simulink library "dsparch2"  (Simulink 3.00)
values from neighbouring files (symbols this model uses):
  h = h./max(h)*0.75    [dspfdes.m]    (also in dspfwiz.m = fdatool(opts); sdspfscope.m = fig_data.menu.memory)
undefined symbols (not defined in the file or in its folder): fchans
libraries: dspbuff2 x4, dspxfrm2 x4, dspbdsp2 x1
settings Model: Creator=szlotkin  LastModifiedBy=jeff

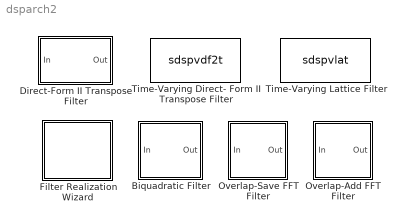
== system dsparch2 ==
  Biquadratic Filter : Subsystem  mask(Biquadratic Filter){sos=[0.0864663705046504 0.172963265055902 0.0864691222801249 1 -0.835073472386969 0.180972230227646;0.0910631887324868 0.184433970597206 0.0934004367730367 1 -0.890597579638043 0.259495175740772;0.10515199960233 0.210266887507767 0.105148652679738 1 -1.0153398584545 0.43590739824434;0.13033445611126 0.257366152017378 0.127072973655515 1 -1.24277336269468 0.75754694447883], ic=0, frame=off, nchans=1}
      mask prompts: sos "SOS matrix:"; ic "Initial conditions:"; frame "Frame-based inputs"; nchans "Number of channels:"
      mask help:
      | Direct-Form II Transpose implementation of second-order (biquadratic) IIR filter sections.  Coefficients must be expressed using an Mx6 second-order section (SOS) matrix.  The number of second-order sections (M) appears in the lower-right corner of the icon.
      |
      | See "ss2sos" for more information on SOS matrices.
      mask init:
      | [x,y,s]=dspblkbiquad('icon',sos);
      | [h,fchans]=dspblkbiquad('init',sos,frame,nchans);
      mask Help: web(dspbhelp);
      mask CallbackString: ||dspblkbiquad|
      mask Display:
      | plot(x,y);
      | text(.975,0.1,s,'horiz','right');
      | text(0.1,.9,'BiQuad')
  Direct-Form II Transpose Filter : Subsystem  mask(Direct-Form II Transpose Filter){num=[1 2], den=1, ic=0, frame=off, numCHANS=1}
      mask prompts: num "Numerator:"; den "Denominator:"; ic "Initial conditions:"; frame "Frame-based inputs"; numCHANS "Number of channels:"
      mask help:
      | Independently filters each channel of input over time using a Direct-Form II Transpose  implementation.  Initial conditions are interpreted in the same manner as MATLAB's "filter" command.
      |
      | For frame-based processing, each column of the input matrix represents one frame of data from a single channel.
      mask init:
      | [x,y] = dspblkdf2t('icon',num,den);
      | if strcmp(frame,'off'), numCHANS=-1; end
      | [num,den] = dspblkdf2t('design',num,den);
      mask Help: web(dspbhelp);
      mask CallbackString: |||dspblkdf2t|
      mask Display:
      | plot(x,y);
      | text(0.5,.85,'DF2T','horiz','center');
  Filter Realization Wizard : Subsystem  mask(Filter Realization Wizard){}
      mask help: Automatically construct filter realizations with specific architectures, using sum, gain, and delay blocks.
      mask init:
      | xw=[NaN 0.8 0.8 NaN 0.687 0.743 NaN 0.64 0.72 NaN 0.687 0.743 NaN 0.8 0.8 NaN 0.913 0.857 NaN 0.96 0.88 NaN 0.808 0.792 0.961 0.978 0.808 NaN 0.825 0.808 NaN 0.961 0.944];
      | yw=[NaN 0.64 0.72 NaN 0.687 0.743 NaN 0.8 0.8 NaN 0.913 0.857 NaN 0.96 0.88 NaN 0.913 0.857 NaN 0.8 0.8 NaN 0.808 0.792 0.622 0.639 0.808 NaN 0.792 0.775 NaN 0.656 0.639];
      | 
      | xl = [.1 .7 NaN .3 .3 NaN .7 .7 NaN .3 .3 NaN .7 .7 NaN .3 .9];
      | yl = [.8 .8 NaN .8 .6 NaN .8 .6 NaN .4 .2 NaN .4 .13 NaN .2 .2];
      | xz = [.46 .54 .46 NaN .54 .59 .54 .59 NaN .61 .64 NaN .67 .67];
      | yz = [.84 .8  .76 NaN .92 .92 .86 .86 NaN .93 .93 NaN .97 .89];
      | xg = [.21 .39 .3 .21 NaN .61 .79 .7 .61];
      | yg = [.6  .6  .4 .6  NaN .6  .6  .4 .6];
      | t=(0:12)/12*2*pi;
      | xs = .07*cos(t)+.7;
      | ys = .07*sin(t)+.2;
      settings: OpenFcn=dspfwiz
      mask Help: web(dspbhelp);
      mask Display:
      | plot([[xl NaN xz NaN xg NaN xs NaN]*.9-.075 xw],
      | [[yl NaN yz NaN yg NaN ys NaN]*.9-.1 yw]);
  Overlap-Add FFT Filter : Subsystem  mask(Overlap-Add FFT Filter){Nfft=64, h=fir1(20,0.1)}
      mask prompts: Nfft "FFT size:"; h "FIR coefficients:"
      mask help: FFT based filtering using the overlap-add algorithm.
      mask init:
      | M = length(h); N=2.^nextpow2(Nfft); L=N-M+1;
      | H = freqz(h,1,N,'whole');
      mask Help: web(dspbhelp);
      mask Display:
      | disp('Overlap\nAdd');
      | ... plot(log10(abs(H(1:(N/2)))))
  Overlap-Save FFT Filter : Subsystem  mask(Overlap-Save FFT Filter){nfft_in=64, h=fir1(20,0.1)}
      mask prompts: nfft_in "FFT size:"; h "FIR coefficients:"
      mask help: FFT based filtering using the overlap-save algorithm.
      mask init:
      | nfft = 2.^nextpow2(nfft_in);
      | n = length(h); H = freqz(h,1,nfft,'whole');
      mask Help: web(dspbhelp);
      mask Display:
      | disp('Overlap\nSave');
      | ... plot(log10(abs(H(1:(nfft/2)))))
  Time-Varying Lattice Filter : S-Function  FunctionName=sdspvlat  Parameters=ARMA, ic, numCHANS, FiltPerFrame  PortCounts=[]  SFunctionModules=''  mask(Time-Varying Lattice Filter){ARMA=All-Zero (MA), ic=0, frame=off, numCHANS=1, FiltPerFrame=One Filter Per Sample Time}
      mask prompts: ARMA "Filter type:"; ic "Initial conditions:"; frame "Frame-based inputs"; numCHANS "Number of channels:"; FiltPerFrame "Filter update rate:"
      mask help:
      | Independently filters each channel of input over time using a Lattice implementation.  Filter coefficients can vary over time.
      |
      | For frame-based processing, multiple data channels may be passed as a frame matrix, with one channel per column.  The filter update rate is selectable.
      mask init:
      | [x,y,s] = dspblkvlat(ARMA);
      | if strcmp(frame,'off') numCHANS = -1; end
      mask Help: web(dspbhelp);
      mask StyleString: popup(All-Zero (MA)|All-Pole (AR)),edit,checkbox,edit,popup(One Filter Per Sample Time|One Filter Per Frame Time)
      mask CallbackString: ||dspblkvlat||
      mask Display:
      | plot(x,y);
      | port_label('input',1,'In');
      | port_label('output',1,'Out');
      | port_label('input',s.i1,s.s1);
      | port_label('input',s.i2,s.s2);
  Time-Varying Direct- Form II Transpose Filter : S-Function  FunctionName=sdspvdf2t  Parameters=NumDen, ic, filtCheck,numCHANS, FiltPerFrame  PortCounts=[]  SFunctionModules=''  mask(Time-Varying Direct-Form II Transpose Filter){NumDen=Pole-Zero (IIR), ic=0, filtCheck=on, frame=off, numCHANS=1, FiltPerFrame=One Filter Per Sample Time}
      mask prompts: NumDen "Filter type:"; ic "Initial conditions:"; filtCheck "Support non-normalized filters"; frame "Frame-based inputs"; numCHANS "Number of channels:"; FiltPerFrame "Filter update rate:"
      mask help:
      | Independently filters each channel of input over time using a Direct-Form II Transpose implementation.  Filter coefficients can vary over time.
      |
      | Initial conditions are interpreted in the same manner as MATLAB's "filter" command.  However, this time-varying filter uses a different normalization scheme and the initial conditions and internal filter states are not equivalent to those from "filter" if the first denominator coefficient is not 1.0.   If "Support non-normalized filters" is deselected, the leading denominator coefficient is assumed to be 1.0.
      |
      | For frame-based processing, multiple data channels may be passed as a frame matrix, with one channel per column.  The filter update rate is selectable.
      mask init:
      | s = dspblkvdf2t(NumDen);
      | if strcmp(frame,'off') numCHANS = -1; end
      mask Help: web(dspbhelp);
      mask StyleString: popup(Pole-Zero (IIR)|All-Zero (FIR)|All-Pole (AR)),edit,checkbox,checkbox,edit,popup(One Filter Per Sample Time|One Filter Per Frame Time)
      mask CallbackString: |||dspblkvdf2t||
      mask Display:
      | text(0.5,0.85,s.icon,'horiz','center');
      | plot(s.x, s.y);
      | port_label('input',1,'In');
      | port_label('output',1,'Out');
      | port_label('input',s.i1,s.s1);
      | port_label('input',s.i2,s.s2);

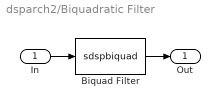
== system dsparch2/Biquadratic Filter ==
  In : Inport  Port=1  PortWidth=-1  SampleTime=-1  DataType=auto
      settings: SignalType=auto
  Biquad Filter : S-Function  FunctionName=sdspbiquad  Parameters=h,ic,fchans  PortCounts=[]  SFunctionModules=''
  Out : Outport  Port=1  InitialOutput=0
  wires:
  In/1 -> Biquad Filter/1
  Biquad Filter/1 -> Out/1

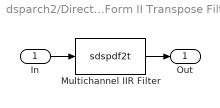
== system dsparch2/Direct-Form II Transpose Filter ==
  In : Inport  Port=1  PortWidth=-1  SampleTime=-1  DataType=auto
      settings: SignalType=auto
  Multichannel IIR Filter : S-Function  FunctionName=sdspdf2t  Parameters=num,den,ic,numCHANS  PortCounts=[]  SFunctionModules=''
  Out : Outport  Port=1  InitialOutput=0
  wires:
  Multichannel IIR Filter/1 -> Out/1
  In/1 -> Multichannel IIR Filter/1

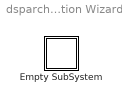
== system dsparch2/Filter Realization Wizard ==
  Empty SubSystem : Subsystem

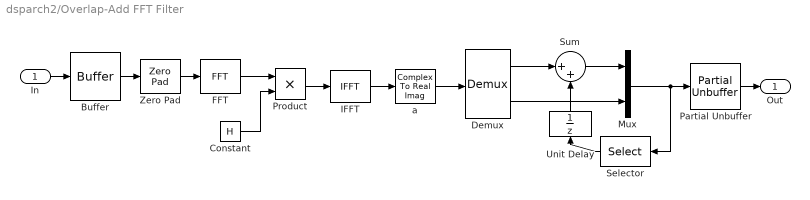
== system dsparch2/Overlap-Add FFT Filter ==
  In : Inport  Port=1  PortWidth=-1  SampleTime=-1  DataType=auto
      settings: SignalType=auto
  Buffer : dspbuff2/Buffer  N=L  V=0  ic=0
  Constant : Constant  Value=H
  Demux : Demux  Outputs=[M-1 L]
  FFT : dspxfrm2/FFT  nchans=1
  IFFT : dspxfrm2/IFFT  mode=Complex  cs_in=off  nchans=1
  Mux : Mux  Inputs=2
  Partial Unbuffer : dspbuff2/Partial Unbuffer  N=N  N1=1  N2=L  ic=0  num_chans=1
  Product : Product  Inputs=2  SaturateOnIntegerOverflow=on
  Selector : Selector  Orientation=left  Elements=[(N-M+2):N]  InputPortWidth=N
  Sum : Sum  Inputs=|++  SaturateOnIntegerOverflow=on
  Unit Delay : UnitDelay  Orientation=up  X0=0  SampleTime=-1
  Zero Pad : dspbdsp2/Zero Pad  pad=N  trunc=on  nchans=1
  a : ComplexToRealImag  Output=Real
  Out : Outport  Port=1  InitialOutput=0
  wires:
  Sum/1 -> Mux/1
  Demux/1 -> Sum/1
  Unit Delay/1 -> Sum/2
  Demux/2 -> Mux/2
  Selector/1 -> Unit Delay/1
  Partial Unbuffer/1 -> Out/1
  Mux/1 -> Partial Unbuffer/1, Selector/1
  In/1 -> Buffer/1
  Product/1 -> IFFT/1
  Constant/1 -> Product/2
  FFT/1 -> Product/1
  Buffer/1 -> Zero Pad/1
  Zero Pad/1 -> FFT/1
  IFFT/1 -> a/1
  a/1 -> Demux/1

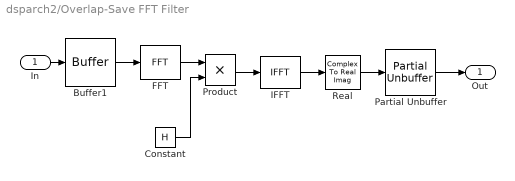
== system dsparch2/Overlap-Save FFT Filter ==
  In : Inport  Port=1  PortWidth=-1  SampleTime=-1  DataType=auto
      settings: SignalType=auto
  Buffer1 : dspbuff2/Buffer  N=nfft  V=n-1  ic=0
  Constant : Constant  Value=H
  FFT : dspxfrm2/FFT  nchans=1
  IFFT : dspxfrm2/IFFT  mode=Complex  cs_in=off  nchans=1
  Partial Unbuffer : dspbuff2/Partial Unbuffer  N=nfft  N1=n  N2=nfft  ic=0  num_chans=1
  Product : Product  Inputs=2  SaturateOnIntegerOverflow=on
  Real : ComplexToRealImag  Output=Real
  Out : Outport  Port=1  InitialOutput=0
  wires:
  In/1 -> Buffer1/1
  FFT/1 -> Product/1
  Constant/1 -> Product/2
  Product/1 -> IFFT/1
  Buffer1/1 -> FFT/1
  Partial Unbuffer/1 -> Out/1
  IFFT/1 -> Real/1
  Real/1 -> Partial Unbuffer/1

== system dsparch2/Filter Realization Wizard/Empty SubSystem ==
